simulink model "sendDataToXplane"  (R2018a)
settings: Solver=VariableStepAuto  StartTime=0.0  StopTime=inf  FixedStep=2/100  RelTol=1e-3  EnableMultiTasking=on
libraries: etargetslib x1, sldrtlib x1, dspnetwork x1
settings Model: Creator=Flight Test Lab  LastModifiedBy=Flight Test Lab
settings SolverCC: ConcurrentTasks=on  AutoInsertRateTranBlk=on
settings DataIOCC: SaveFormat=StructureWithTime
settings OptimizationCC: BlockReduction=off  DefaultUnderspecifiedDataType=single  OptimizeBlockIOStorage=off  BufferReuse=off  GlobalBufferReuse=off  ExpressionFolding=off  LocalBlockOutputs=off  OptimizeDataStoreBuffers=off  BusAssignmentInplaceUpdate=off
settings RTWCC: Description=Generic Real-Time Target  RTWCompilerOptimization=on
settings CodeAppCC: MaxIdLength=95
settings GRTTargetCC: TargetLangStandard=C89/C90 (ANSI)

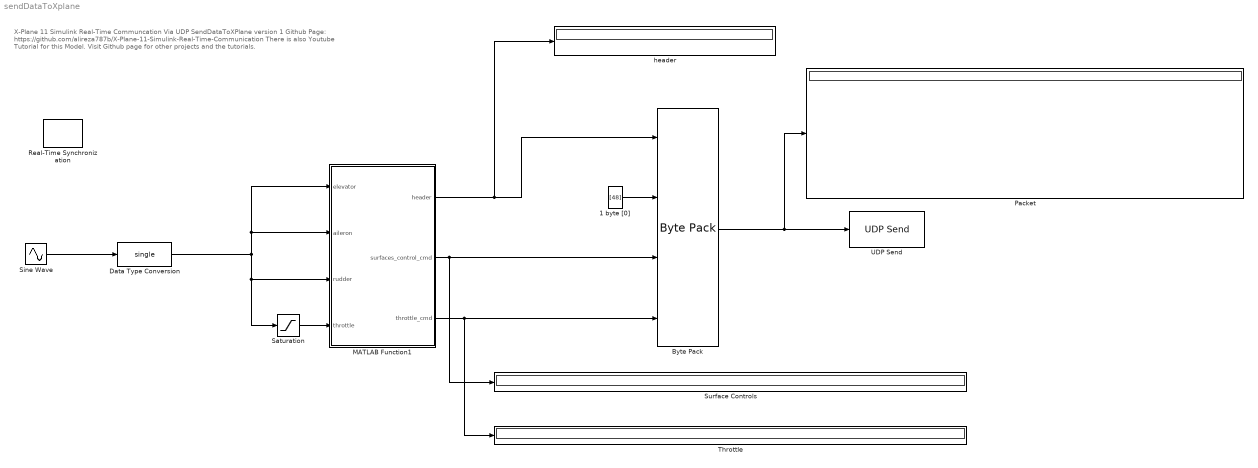
== system sendDataToXplane ==
  note: X-Plane 11 Simulink Real-Time Communcation Via UDP
      | SendDataToXPlane version 1
      | Github Page:
      | https://github.com/alireza787b/X-Plane-11-Simulink-Real-Time-Communication
      | There is also Youtube Tutorial for this Model.
      | Visit Github page for other projects and the tutorials.
  1 byte [0] : Constant  Value=[48]  OutDataTypeStr=uint8
  Byte Pack : etargetslib/Byte Pack  datatypes={'uint8','uint8','single','single'}  byteAlign=1
  Data Type Conversion : DataTypeConversion  OutDataTypeStr=single
  MATLAB Function1 : MATLAB Function  TreatAsAtomicUnit=on
  Packet : Display
  Real-Time Synchronization : sldrtlib/Real-Time Synchronization  SampleTime=.02  MaxMissedTicks=10  ShowMissedTicks=off  YieldWhenWaiting=off
  Saturation : Saturate  UpperLimit=1  LowerLimit=0
  Sine Wave : Sin  SampleTime=0
  Surface Controls : Display
  Throttle : Display
  UDP Send : dspnetwork/UDP Send  remoteURL='127.0.0.1'  remotePort=49000  localURL='0.0.0.0'  localPortSource=Automatically determine  localPort=-1  sampletime=-1  blockPlatform=[]  separateLengthPort=0
      settings: SourceProductName=DSP System Toolbox  SourceProductBaseCode=DS
  header : Display
  wires:
  Byte Pack/1 -> UDP Send/1, Packet/1
  Data Type Conversion/1 -> Saturation/1, MATLAB Function1/3(rudder), MATLAB Function1/2(aileron), MATLAB Function1/1(elevator)
  MATLAB Function1/3(throttle_cmd) -> Throttle/1, Byte Pack/4
  1 byte [0]/1 -> Byte Pack/2
  MATLAB Function1/1(header) -> Byte Pack/1, header/1
  MATLAB Function1/2(surfaces_control_cmd) -> Surface Controls/1, Byte Pack/3
  Sine Wave/1 -> Data Type Conversion/1
  Saturation/1 -> MATLAB Function1/4(throttle)

== matlab function sendDataToXplane/MATLAB Function1 ==
  data: elevator input; header output uint8; surfaces_control_cmd output; aileron input single; rudder input single; throttle input; throttle_cmd output single
function [header,surfaces_control_cmd,throttle_cmd] = fcn(elevator, aileron, rudder, throttle) 
header =[uint8(68) uint8(65) uint8(84) uint8(65)];
No_Comand = single(-999);
 %Surface_header = typecast(uint8([uint8(8) uint8(0) uint8(0) uint8(0)]),'single')
surfaces_control_cmd = [1.1210388e-44 elevator aileron rudder No_Comand No_Comand No_Comand No_Comand No_Comand  ];
%Throttle_header = typecast(uint8([uint8(25) uint8(0) uint8(0) uint8(0)]),'single');
throttle_cmd = [3.503246160812043e-44 throttle No_Comand No_Comand No_Comand No_Comand No_Comand No_Comand No_Comand];
end
